simulink model "example_DHWconsumptionEn13203"  (R2016b)
settings: Solver=ode45  StartTime=0.0  StopTime=24*3600  RelTol=1e-3  EnableMultiTasking=on
libraries: carnot x5
settings Model: Creator=drhf  LastModifiedBy=drhf
settings DataIOCC: LimitDataPoints=on  SaveFormat=Array  SignalLoggingSaveFormat=ModelDataLogs
settings OptimizationCC: ExpressionDepthLimit=2147483647  LifeSpan=inf
settings DebuggingCC: UnderspecifiedInitializationDetection=Classic  MergeDetectMultiDrivingBlocksExec=none  SolverPrmCheckMsg=warning  StateNameClashWarn=warning  SFUnexpectedBacktrackingDiag=warning  SFNoUnconditionalDefaultTransitionDiag=warning  SFExecutionAtInitializationDiag=none
settings HardwareCC: ProdBitPerPointer=32  ProdBitPerSizeT=32  ProdBitPerPtrDiffT=32  ProdLargestAtomicFloat=None  ProdIntDivRoundTo=Undefined  ProdEndianess=Unspecified  ProdWordSize=32  ProdHWDeviceType=32-bit Generic
settings ModelReferenceCC: PropagateSignalLabelsOutOfModel=off
settings GRTTargetCC: TargetLangStandard=C89/C90 (ANSI)  GeneratePreprocessorConditionals=Disable all  CombineOutputUpdateFcns=off  GRTInterface=on
settings ConfigComp: CovMetricSettings=dw  CovHtmlReporting=on  CovSaveCumulativeToWorkspaceVar=on  CovSaveSingleToWorkspaceVar=on  CovExternalEMLEnable=off

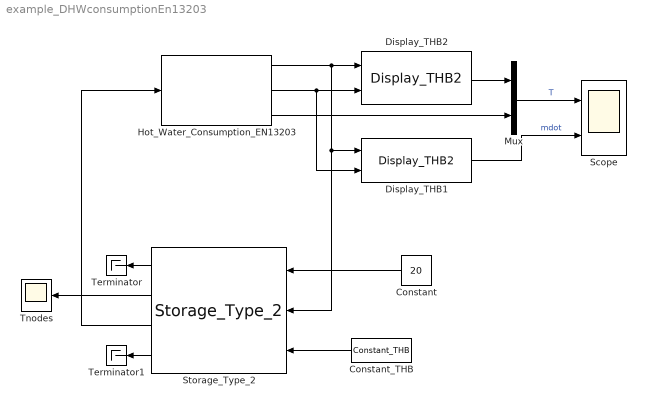
== system example_DHWconsumptionEn13203 ==
  Constant : Constant  Value=20
  Constant_THB : carnot/Source/Simple/Constant_THB  t=40  mdot=0*100/3600  p=1e5  mID=No Pressure Drop  fluid=Water  mix=0  mix2=0  mix3=0  dia=0.02  hgt=0
  Display_THB1 : carnot/Outputs/Display_THB2  t=off  m=on  p=off  id=off  mix=off  d=off
  Display_THB2 : carnot/Outputs/Display_THB2  t=on  m=off  p=off  id=off  mix=off  d=off
  Hot_Water_Consumption_EN13203 : carnot/Load/Hot_Water_Tapping/Applications/Hot_Water_Consumption_EN13203  SystemSampleTime=-1
  Mux : Mux  Inputs=2
  Scope : Scope  NumInputPorts=2
  Storage_Type_2 : carnot/Storage/Thermal/Storage_Type_2  uloss=1  ubot=1  utop=1  cond=1  volume=0.3  dia=0.5  pos=standing cylinder  h_in_chg=0.5  h_out_chg=0.1  ua0=80  uam=0.2  uat=0.5  dplin_chg=100  dpqua_chg=100  h_in=0  h_out=1  dplin=10  dpqua=10  t0=[10:5:55]  nodes=10  mpoints=10
  Terminator : Terminator
  Terminator1 : Terminator
  Tnodes : Scope
  wires:
  Storage_Type_2/3 -> Hot_Water_Consumption_EN13203/1
  Hot_Water_Consumption_EN13203/1 -> Display_THB1/1, Storage_Type_2/2, Display_THB2/1
  Hot_Water_Consumption_EN13203/2 -> Display_THB2/2, Display_THB1/2
  Display_THB2/1 -> Mux/1
  Hot_Water_Consumption_EN13203/3 -> Mux/2
  Mux/1 -> Scope/1  "T"
  Display_THB1/1 -> Scope/2  "mdot"
  Storage_Type_2/1 -> Terminator/1
  Storage_Type_2/4 -> Terminator1/1
  Constant_THB/1 -> Storage_Type_2/3
  Constant/1 -> Storage_Type_2/1
  Storage_Type_2/2 -> Tnodes/1
